simulink model "CthulhuFinalSimulation"  (R2019a)
settings: Solver=FixedStepDiscrete  StartTime=0.0  StopTime=500  FixedStep=dt  RelTol=1e-3
InitFcn:
  | clc
  | clear
  | 
  | timedelay = 0.05; %input lag, s
  | 
  | m = 2.5;
  | I = [0.034,  0.00008985,      -0.004;
  |         0.00008985,       0.075, -0.00000266;
  |       -0.004, -0.00000266,       0.102]; %kg m^2
  | 
  | L_p = 0.54; %length of pontoon, m
  | d_p = 0.1; %diameter of pontoon, m
  | V_p = 0.002536; %volume of pontoon, m
  | w_c = 0.347; %distance between pontoons, m
  | Zcm = 0.0; %height of cm wrt pontoons, m
  | 
  | wave_amp = 0.005; %amplitude of waves, m
  | f = 1.5; %freq of waves, Hz
  | 
  | Ayz = 0.002; %Area projected onto yz plane
  | Axz = 0.002; %Area projected onto xz plane
  | Axy = 0.005; %Area projected onto xy plane
  | Cdx = 2.2;
  | Cdy = 2.2;
  | Cdz = 2.2;
  | 
  | Iinv = I^-1;
  | dt = 0.005;
  | dtsim = 1/25;
  | dtdata = 0.01;
  | dtcontrol = 0.1;
  | timeseed = clock;
  | timeseed = round(timeseed(6));
  | wo = [0;0;0];
  | Ho = [0;0;0];
  | ro = [63;-31.5;d_p/2+0.3];
  | vo = [0;0;0];
  | qTarget = [1;0;0;0];
  | R = 0.1;
  | P = 0.0001;
  | Y = 0;
  | qo = [cos(R/2)*cos(P/2)*cos(Y/2)-sin(R/2)*sin(P/2)*sin(Y/2);
  |          sin(R/2)*cos(P/2)*cos(Y/2)+cos(R/2)*sin(P/2)*sin(Y/2);
  |          cos(R/2)*sin(P/2)*cos(Y/2)-sin(R/2)*cos(P/2)*sin(Y/2);
  |          sin(R/2)*sin(P/2)*cos(Y/2)+cos(R/2)*cos(P/2)*sin(Y/2)];
  | 
  | g = 9.80248;
  | rho = 997;
  | 
  | myworld = vrworld('CthulhuAssembly.wrl');
  | open(myworld);
  | set(0,'Units','pixels');
  | scnsize = get(0,'ScreenSize');
  | f1 = vrfigure(myworld,[1 80 scnsize(3)/2 scnsize(4)/2]);
  | set(f1,'Viewpoint','BodyView')
  | 
  | %pause(10)
StopFcn:
  | %plots_manual_control
undefined symbols (not defined in the file or in its folder): DiscIntNeverNeededParam
libraries: sharedtransform x5, vrlib x5, aerolibutil x3, aerolibanimutils x1, simulink x1
settings Model: Creator=washickb  LastModifiedBy=underwj5
settings DataIOCC: ReturnWorkspaceOutputs=off
settings DebuggingCC: ArithmeticOperatorsInVariantConditions=warning
settings SFSimCC: SimUseLocalCustomCode=off
settings RTWCC: RTWUseLocalCustomCode=off

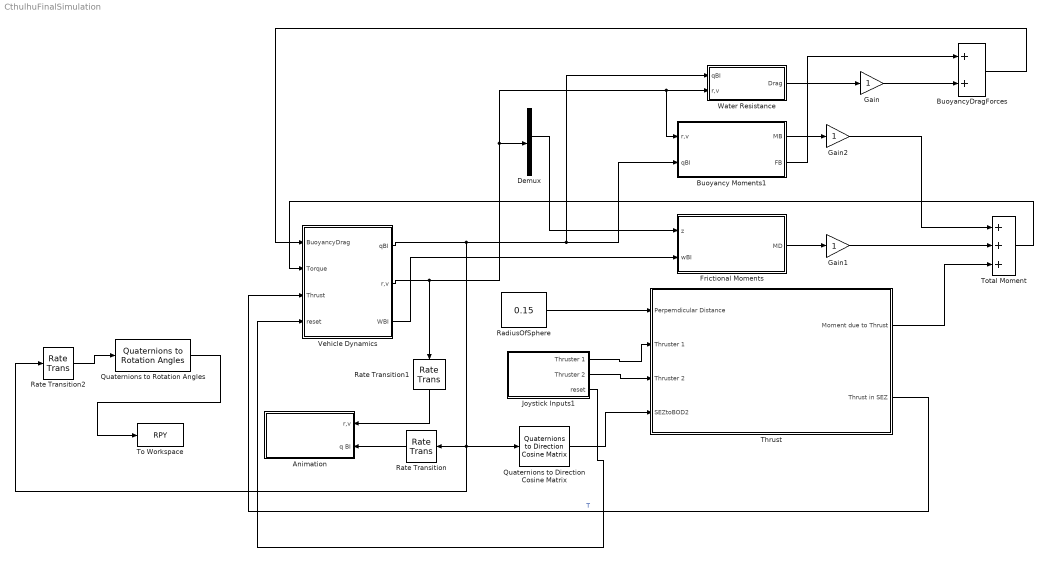
== system CthulhuFinalSimulation ==
  Animation : Subsystem
  Buoyancy Moments1 : Subsystem
  BuoyancyDragForces : Sum  Inputs=2
  Demux : Demux  Outputs=6
  Frictional Moments : Subsystem
  Gain : Gain
  Gain1 : Gain
  Gain2 : Gain
  Joystick Inputs1 : Subsystem
  Quaternions to Direction Cosine Matrix : sharedtransform/Quaternions to  Direction Cosine Matrix  aMode=aMode
      settings: SourceProductName=Aerospace Blockset  SourceProductBaseCode=AE
  Quaternions to Rotation Angles : sharedtransform/Quaternions to Rotation Angles  rotationOrder=XYZ  aMode=aMode
      settings: SourceProductBaseCode=AE
  RadiusOfSphere : Constant  Value=0.15
  Rate Transition : RateTransition  InitialCondition=qo  OutPortSampleTime=dtsim
  Rate Transition1 : RateTransition  InitialCondition=[ro;vo]  OutPortSampleTime=dtsim
  Rate Transition2 : RateTransition  InitialCondition=qo  OutPortSampleTime=dtdata
  "Thrust " : Subsystem
  To Workspace : ToWorkspace  VariableName=RPY  SaveFormat=Structure With Time  SampleTime=-1
  Total Moment : Sum  Inputs=+++
  Vehicle Dynamics : Subsystem
  Water Resistance : Subsystem
  wires:
  Vehicle Dynamics/2(r,v) -> Demux/1, Buoyancy Moments1/1(r,v), Water Resistance/2(r,v), Rate Transition1/1
  Vehicle Dynamics/1(qBI) -> Quaternions to Direction Cosine Matrix/1, Rate Transition2/1, Rate Transition/1, Water Resistance/1(qBI), Buoyancy Moments1/2(qBI)
  Rate Transition1/1 -> Animation/1(r,v)
  Rate Transition/1 -> Animation/2(q BI)
  Quaternions to Direction Cosine Matrix/1 -> "Thrust "/4(SEZtoBOD2)
  "Thrust "/1("Moment due to Thrust ") -> Total Moment/3
  Joystick Inputs1/2(Thruster 2) -> "Thrust "/3(Thruster 2)
  Joystick Inputs1/1(Thruster 1) -> "Thrust "/2(Thruster 1)
  RadiusOfSphere/1 -> "Thrust "/1(Perpemdicular Distance)
  Quaternions to Rotation Angles/1 -> To Workspace/1
  Vehicle Dynamics/3(WBI) -> Frictional Moments/2(wBI)
  Rate Transition2/1 -> Quaternions to Rotation Angles/1
  Total Moment/1 -> Vehicle Dynamics/2(Torque)
  "Thrust "/2(Thrust in SEZ) -> Vehicle Dynamics/3(Thrust)  "T"
  Buoyancy Moments1/1(MB) -> Gain2/1
  Demux/3 -> Frictional Moments/1(z)
  Frictional Moments/1("MD ") -> Gain1/1
  Water Resistance/1(Drag) -> Gain/1
  BuoyancyDragForces/1 -> Vehicle Dynamics/1(BuoyancyDrag)
  Gain/1 -> BuoyancyDragForces/2
  Gain1/1 -> Total Moment/2
  Gain2/1 -> Total Moment/1
  Buoyancy Moments1/2(FB) -> BuoyancyDragForces/1
  Joystick Inputs1/3(reset) -> Vehicle Dynamics/4(reset)

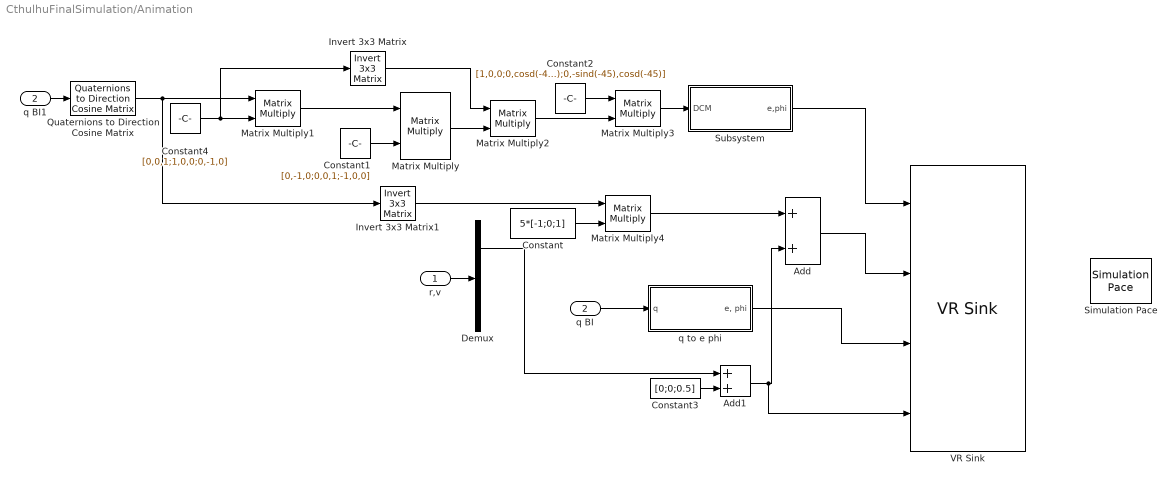
== system CthulhuFinalSimulation/Animation ==
  r,v : Inport
  q BI : Inport  Port=2
  Add : Sum
  Add1 : Sum
  Constant : Constant  Value=5*[-1;0;1]
  Constant1 : Constant  Value=[0,-1,0;0,0,1;-1,0,0]
  Constant2 : Constant  Value=[1,0,0;0,cosd(-45),sind(-45);0,-sind(-45),cosd(-45)]
  Constant3 : Constant  Value=[0;0;0.5]
  Constant4 : Constant  Value=[0,0,1;1,0,0;0,-1,0]
  Demux : Demux  Outputs=[3 3]
  Invert 3x3 Matrix : aerolibutil/Invert  3x3 Matrix
  Invert 3x3 Matrix1 : aerolibutil/Invert  3x3 Matrix
  Matrix Multiply{,1..4} (5 alike) : Product  Multiplication=Matrix(*)
  Quaternions to Direction Cosine Matrix : sharedtransform/Quaternions to  Direction Cosine Matrix  aMode=aMode
      settings: SourceProductName=Aerospace Blockset  SourceProductBaseCode=AE
  Simulation Pace : aerolibanimutils/Simulation Pace  SimulationPace=1  SleepMode=Auto  OutputPaceError=off  SampleTime=dt
  Subsystem : Subsystem
  VR Sink : vrlib/VR Sink  InstantiateOnLoad=on  SampleTime=0.1  ViewEnable=on  RemoteChange=off  RemoteView=off  FieldsWritten=BodyView.orientation.4.1.1.double#BodyView.position.3.1.1.double#Cthulhu.rotation.4.1.1.double#Cthulhu.translation.3.1.1.double  WorldFileName=CthulhuAssembly.wrl  AutoView=off  VideoDimensions=[]  AllowVariableSize=off
      settings: SourceProductName=Simulink
  q BI1 : InportShadow  Port=2
  q to e phi : Subsystem
  wires:
  r,v/1 -> Demux/1
  q BI/1 -> q to e phi/1("q ")
  Demux/1 -> Add1/1
  Constant1/1 -> Matrix Multiply/2
  Quaternions to Direction Cosine Matrix/1 -> Invert 3x3 Matrix1/1, Matrix Multiply1/1
  Add1/1 -> VR Sink/4, Add/2
  Constant3/1 -> Add1/2
  Constant/1 -> Matrix Multiply4/2
  q BI1/1 -> Quaternions to Direction Cosine Matrix/1
  Matrix Multiply2/1 -> Matrix Multiply3/2
  Matrix Multiply1/1 -> Matrix Multiply/1
  Constant4/1 -> Invert 3x3 Matrix/1, Matrix Multiply1/2
  Matrix Multiply/1 -> Matrix Multiply2/2
  Invert 3x3 Matrix/1 -> Matrix Multiply2/1
  Constant2/1 -> Matrix Multiply3/1
  Matrix Multiply3/1 -> Subsystem/1(DCM)
  Matrix Multiply4/1 -> Add/1
  Invert 3x3 Matrix1/1 -> Matrix Multiply4/1
  Subsystem/1(e,phi) -> VR Sink/1
  Add/1 -> VR Sink/2
  q to e phi/1("e, phi") -> VR Sink/3

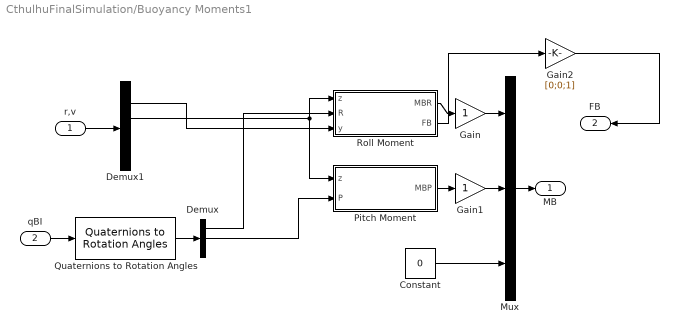
== system CthulhuFinalSimulation/Buoyancy Moments1 ==
  r,v : Inport
  qBI : Inport  Port=2
  Constant : Constant  Value=0
  Demux : Demux  Outputs=3
  Demux1 : Demux  Outputs=6
  Gain : Gain
  Gain1 : Gain
  Gain2 : Gain  Gain=[0;0;1]
  Mux : Mux  Inputs=3
  Pitch Moment : Subsystem
  Quaternions to Rotation Angles : sharedtransform/Quaternions to Rotation Angles  rotationOrder=XYZ  aMode=aMode
      settings: SourceProductBaseCode=AE
  Roll Moment : Subsystem
  MB : Outport
  FB : Outport  Port=2
  wires:
  Constant/1 -> Mux/3
  Mux/1 -> MB/1
  Pitch Moment/1(MBP) -> Gain1/1
  Roll Moment/1(MBR) -> Gain/1
  qBI/1 -> Quaternions to Rotation Angles/1
  Quaternions to Rotation Angles/1 -> Demux/1
  Demux/1 -> Roll Moment/2(R)
  Demux/2 -> Pitch Moment/2(P)
  Gain/1 -> Mux/1
  Gain1/1 -> Mux/2
  Roll Moment/2(FB) -> Gain2/1
  Gain2/1 -> FB/1
  r,v/1 -> Demux1/1
  Demux1/3 -> Pitch Moment/1(z), Roll Moment/1(z)
  Demux1/2 -> Roll Moment/3(y)

== system CthulhuFinalSimulation/Frictional Moments ==
  z : Inport
  wBI : Inport  Port=2
  Add : Sum  Inputs=+---
  Constant : Constant  Value=Zcm
  Constant1 : Constant  Value=d_p/2
  Constant2 : Constant  Value=.05
  If : If  IfExpression=u1 < 0
  If Action Subsystem : Subsystem  TreatAsAtomicUnit=on
  Merge : Merge
  Subsystem : Subsystem
  "MD " : Outport
  wires:
  If/1 -> Subsystem/Action  "z<d_p"
  If/2 -> If Action Subsystem/Action
  Subsystem/1(MD) -> Merge/2
  If Action Subsystem/1(Out1) -> Merge/1
  Merge/1 -> "MD "/1
  z/1 -> Add/1
  Constant/1 -> Add/2
  Constant1/1 -> Add/3
  Add/1 -> If/1
  Constant2/1 -> Add/4
  wBI/1 -> Subsystem/1(wBI)

== system CthulhuFinalSimulation/Joystick Inputs1 ==
  Demux : Demux  Outputs=5
  Demux1 : Demux  Outputs=10
  Gain1 : Gain  Gain=-1
  Gain2 : Gain  Gain=-1
  Joystick Input : vrlib/Joystick Input  joyid=1  adjustports=on  forcefeed=off
      settings: SourceProductName=Simulink
  Stop Simulation : Stop
  Subsystem : Subsystem
  Subsystem2 : Subsystem
  Thruster 1 : Outport
  Thruster 2 : Outport  Port=2
  reset : Outport  Port=3
  wires:
  Demux/2 -> Gain1/1
  Gain1/1 -> Subsystem/1(pad y)  "pad y"
  Joystick Input/1 -> Demux/1
  Gain2/1 -> Subsystem2/1(pad y)  "pad y"
  Demux/5 -> Gain2/1
  Subsystem2/1(thrust) -> Thruster 2/1
  Subsystem/1(thrust) -> Thruster 1/1
  Joystick Input/2 -> Demux1/1
  Demux1/8 -> reset/1
  Demux1/1 -> Stop Simulation/1

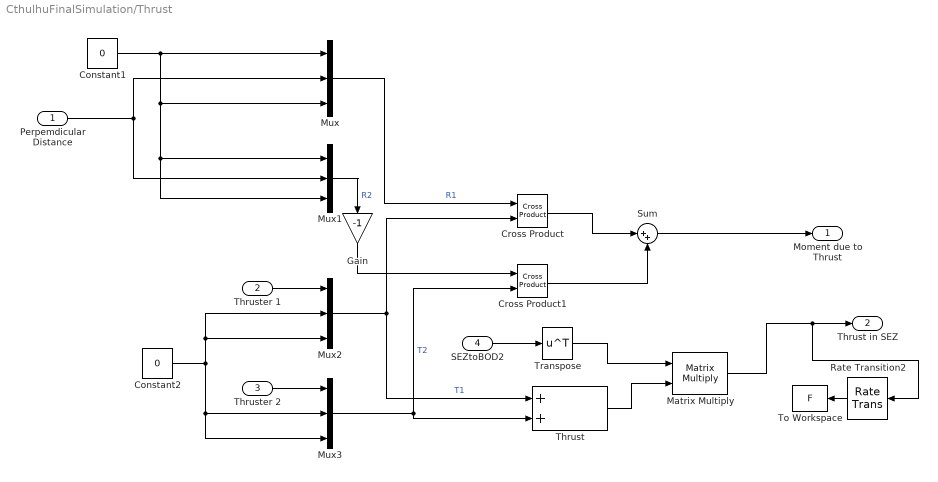
== system CthulhuFinalSimulation/Thrust  ==
  Perpemdicular Distance : Inport
  Thruster 1 : Inport  Port=2
  Thruster 2 : Inport  Port=3
  SEZtoBOD2 : Inport  Port=4
  Constant1 : Constant  Value=0
  Constant2 : Constant  Value=0
  Cross Product : vrlib/Utilities/Cross Product
      settings: SourceProductName=Simulink
  Cross Product1 : vrlib/Utilities/Cross Product
      settings: SourceProductName=Simulink
  Gain : Gain  Gain=-1
  Matrix Multiply : Product  Multiplication=Matrix(*)
  Mux{,1..3} (4 alike) : Mux  Inputs=3
  Rate Transition2 : RateTransition  InitialCondition=[0;0;0]  OutPortSampleTime=dtdata
  Sum : Sum  Inputs=|++
  Thrust : Sum  Inputs=2
  To Workspace : ToWorkspace  VariableName=F  SaveFormat=Structure With Time  SampleTime=-1
  Transpose : Math  Operator=transpose  SaturateOnIntegerOverflow=on
  "Moment due to Thrust " : Outport
  Thrust in SEZ : Outport  Port=2
  wires:
  Perpemdicular Distance/1 -> Mux1/2, Mux/2
  Constant1/1 -> Mux/1, Mux1/3, Mux1/1, Mux/3
  Thruster 1/1 -> Mux2/1
  Thruster 2/1 -> Mux3/1
  Constant2/1 -> Mux3/3, Mux3/2, Mux2/3, Mux2/2
  Mux2/1 -> Cross Product/2, Thrust/1  "T1"
  Mux3/1 -> Cross Product1/2, Thrust/2  "T2"
  Mux/1 -> Cross Product/1  "R1"
  Mux1/1 -> Gain/1  "R2"
  Cross Product/1 -> Sum/1
  Cross Product1/1 -> Sum/2
  Sum/1 -> "Moment due to Thrust "/1
  SEZtoBOD2/1 -> Transpose/1
  Transpose/1 -> Matrix Multiply/1
  Thrust/1 -> Matrix Multiply/2
  Matrix Multiply/1 -> Rate Transition2/1, Thrust in SEZ/1
  Gain/1 -> Cross Product1/1
  Rate Transition2/1 -> To Workspace/1

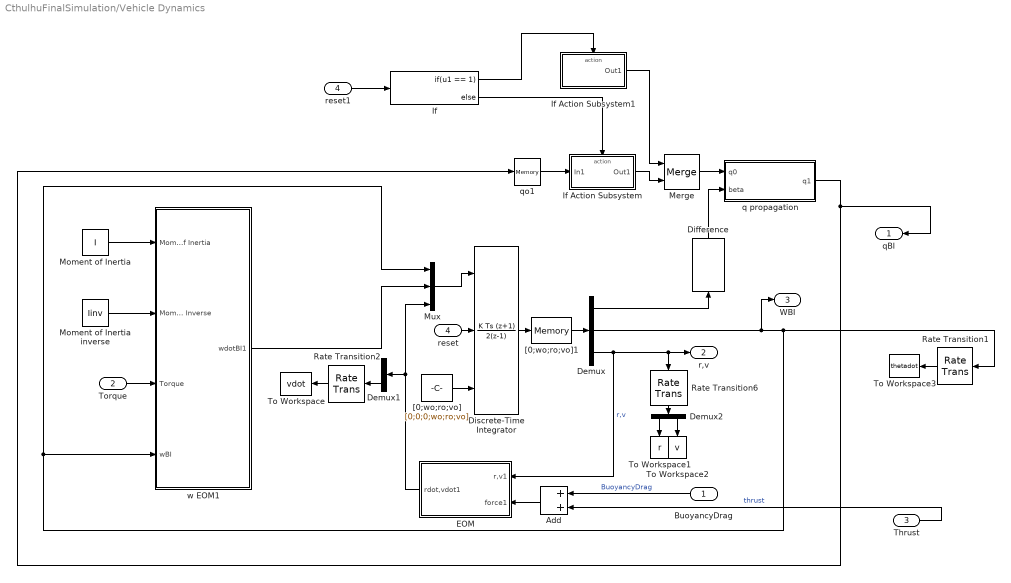
== system CthulhuFinalSimulation/Vehicle Dynamics ==
  BuoyancyDrag : Inport
  Torque : Inport  Port=2
  Thrust : Inport  Port=3
  reset : Inport  Port=4
  Add : Sum
  Demux : Demux  Outputs=[3 3 6]
  Demux1 : Demux  Outputs=2
  Demux2 : Demux  Outputs=2
  Difference : simulink/Discrete/Difference  ICPrevInput=0.0  OutMin=[]  OutMax=[]  OutDataType=fixdt(1, 16)  OutScaling=2^-10  DoSatur=off
  Discrete-Time Integrator : DiscreteIntegrator  IntegratorMethod=Integration: Trapezoidal  ExternalReset=rising  InitialConditionSource=external  SampleTime=dt  ICPrevOutput=DiscIntNeverNeededParam  ICPrevScaledInput=DiscIntNeverNeededParam
  EOM : Subsystem
  If : If  IfExpression=u1 == 1
  If Action Subsystem : Subsystem  TreatAsAtomicUnit=on
  If Action Subsystem1 : Subsystem  TreatAsAtomicUnit=on
  Merge : Merge
  Moment of Inertia : Constant  Value=I
  Moment of Inertia inverse : Constant  Value=Iinv
  Mux : Mux  Inputs=3
  Rate Transition1 : RateTransition  InitialCondition=[0;0;0]  OutPortSampleTime=dtdata
  Rate Transition2 : RateTransition  InitialCondition=[0;0;0]  OutPortSampleTime=dtdata
  Rate Transition6 : RateTransition  InitialCondition=[0;0;0;0;0;0]  OutPortSampleTime=dtdata
  To Workspace : ToWorkspace  VariableName=vdot  SaveFormat=Structure With Time  SampleTime=-1
  To Workspace1 : ToWorkspace  VariableName=r  SaveFormat=Structure With Time  SampleTime=-1
  To Workspace2 : ToWorkspace  VariableName=v  SaveFormat=Structure With Time  SampleTime=-1
  To Workspace3 : ToWorkspace  VariableName=thetadot  SaveFormat=Structure With Time  SampleTime=-1
  "[0;wo;ro;vo]" : Constant  Value=[0;0;0;wo;ro;vo]
  "[0;wo;ro;vo]1" : Memory  InitialCondition=[0;0;0;wo;ro;vo]  InheritSampleTime=on
  q propagation : Subsystem
  qo1 : Memory  InitialCondition=qo
  reset1 : InportShadow  Port=4
  w EOM1 : Subsystem
  qBI : Outport
  r,v : Outport  Port=2
  WBI : Outport  Port=3
  wires:
  Difference/1 -> q propagation/2(beta)
  Moment of Inertia/1 -> w EOM1/1(Moment of Inertia)
  Moment of Inertia inverse/1 -> w EOM1/2(Moment of Inertia Inverse)
  qo1/1 -> If Action Subsystem/1(In1)
  Discrete-Time Integrator/1 -> "[0;wo;ro;vo]1"/1
  Mux/1 -> Discrete-Time Integrator/1
  Demux/3 -> EOM/1(r,v1), r,v/1, Rate Transition6/1  "r,v"
  "[0;wo;ro;vo]1"/1 -> Demux/1
  q propagation/1(q1) -> qo1/1, qBI/1
  Torque/1 -> w EOM1/3(Torque)
  "[0;wo;ro;vo]"/1 -> Discrete-Time Integrator/3
  Demux/1 -> Difference/1
  w EOM1/1(wdotBI1) -> Mux/2
  Demux1/2 -> Rate Transition2/1
  Rate Transition2/1 -> To Workspace/1
  EOM/1(rdot,vdot1) -> Demux1/1, Mux/3
  Thrust/1 -> Add/2  "thrust"
  BuoyancyDrag/1 -> Add/1  "BuoyancyDrag"
  Rate Transition6/1 -> Demux2/1
  Demux2/1 -> To Workspace1/1
  Demux2/2 -> To Workspace2/1
  Add/1 -> EOM/2(force1)
  Demux/2 -> Rate Transition1/1, w EOM1/4(wBI), Mux/1, WBI/1
  Rate Transition1/1 -> To Workspace3/1
  reset/1 -> Discrete-Time Integrator/2
  reset1/1 -> If/1
  If/2 -> If Action Subsystem/Action
  If/1 -> If Action Subsystem1/Action
  Merge/1 -> q propagation/1(q0)
  If Action Subsystem1/1(Out1) -> Merge/1
  If Action Subsystem/1(Out1) -> Merge/2

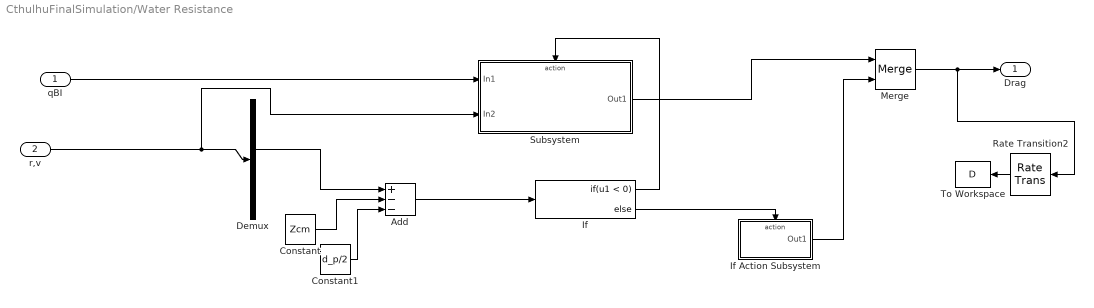
== system CthulhuFinalSimulation/Water Resistance ==
  qBI : Inport
  r,v : Inport  Port=2
  Add : Sum  Inputs=+--
  Constant : Constant  Value=Zcm
  Constant1 : Constant  Value=d_p/2
  Demux : Demux  Outputs=6
  If : If  IfExpression=u1 < 0
  If Action Subsystem : Subsystem  TreatAsAtomicUnit=on
  Merge : Merge
  Rate Transition2 : RateTransition  InitialCondition=[0;0;0]  OutPortSampleTime=dtdata
  Subsystem : Subsystem
  To Workspace : ToWorkspace  VariableName=D  SaveFormat=Structure With Time  SampleTime=-1
  Drag : Outport
  wires:
  qBI/1 -> Subsystem/1(In1)
  r,v/1 -> Subsystem/2(In2), Demux/1
  Constant/1 -> Add/2
  Constant1/1 -> Add/3
  Demux/3 -> Add/1
  Add/1 -> If/1
  If/1 -> Subsystem/Action
  If/2 -> If Action Subsystem/Action
  If Action Subsystem/1(Out1) -> Merge/2
  Subsystem/1(Out1) -> Merge/1
  Merge/1 -> Rate Transition2/1, Drag/1
  Rate Transition2/1 -> To Workspace/1

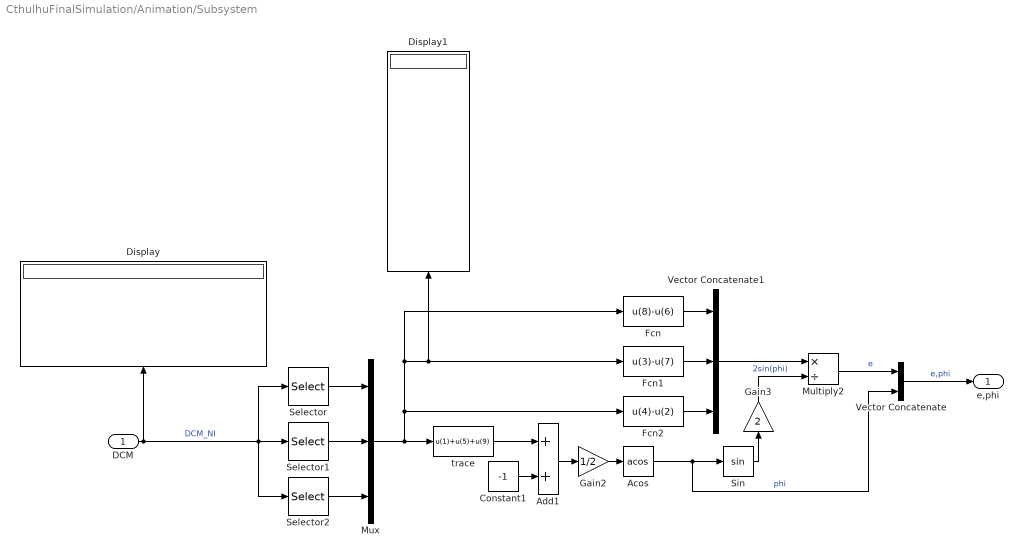
== system CthulhuFinalSimulation/Animation/Subsystem ==
  DCM : Inport
  Acos : Trigonometry  Operator=acos
  Add1 : Sum
  Constant1 : Constant  Value=-1
  Display : Display
  Display1 : Display
  Fcn : Fcn  Expr=u(8)-u(6)
  Fcn1 : Fcn  Expr=u(3)-u(7)
  Fcn2 : Fcn  Expr=u(4)-u(2)
  Gain2 : Gain  Gain=1/2
  Gain3 : Gain  Gain=2
  Multiply2 : Product  Inputs=*/
  Mux : Mux  Inputs=3
  Selector : Selector  NumberOfDimensions=2  InputPortWidth=3  IndexOptions=Select all,Index vector (dialog)  Indices=[1 3],1  OutputSizes=1,1
  Selector1 : Selector  NumberOfDimensions=2  InputPortWidth=3  IndexOptions=Select all,Index vector (dialog)  Indices=[1 3],2  OutputSizes=1,1
  Selector2 : Selector  NumberOfDimensions=2  InputPortWidth=3  IndexOptions=Select all,Index vector (dialog)  Indices=[1 3],3  OutputSizes=1,1
  Sin : Trigonometry
  Vector Concatenate : Concatenate
  Vector Concatenate1 : Concatenate  NumInputs=3
  trace : Fcn  Expr=u(1)+u(5)+u(9)
  e,phi : Outport
  wires:
  Vector Concatenate1/1 -> Multiply2/1
  trace/1 -> Add1/1
  Add1/1 -> Gain2/1
  Vector Concatenate/1 -> e,phi/1  "e,phi"
  Constant1/1 -> Add1/2
  Fcn/1 -> Vector Concatenate1/1
  Gain3/1 -> Multiply2/2  "2sin(phi)"
  Multiply2/1 -> Vector Concatenate/1  "e"
  Sin/1 -> Gain3/1
  Fcn1/1 -> Vector Concatenate1/2
  Acos/1 -> Vector Concatenate/2, Sin/1  "phi"
  Fcn2/1 -> Vector Concatenate1/3
  Gain2/1 -> Acos/1
  Mux/1 -> Fcn2/1, Fcn1/1, Display1/1, Fcn/1, trace/1
  Selector/1 -> Mux/1
  Selector1/1 -> Mux/2
  Selector2/1 -> Mux/3
  DCM/1 -> Selector2/1, Selector/1, Selector1/1, Display/1  "DCM_NI"

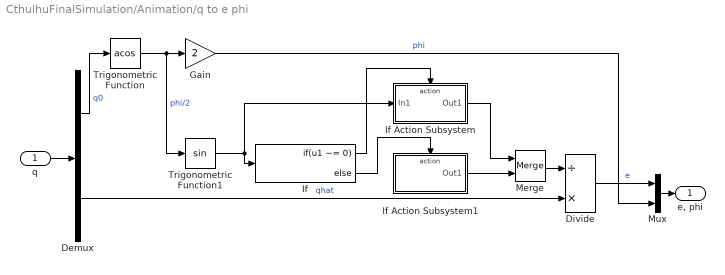
== system CthulhuFinalSimulation/Animation/q to e phi ==
  "q " : Inport
  Demux : Demux  Outputs=[1,3]
  Divide : Product  Inputs=/*
  Gain : Gain  Gain=2
  If : If  IfExpression=u1 ~= 0
  If Action Subsystem : Subsystem  TreatAsAtomicUnit=on
  If Action Subsystem1 : Subsystem  TreatAsAtomicUnit=on
  Merge : Merge
  Mux : Mux  Inputs=2
  Trigonometric Function : Trigonometry  Operator=acos
  Trigonometric Function1 : Trigonometry
  "e, phi" : Outport
  wires:
  Gain/1 -> Mux/2  "phi"
  Demux/1 -> Trigonometric Function/1  "q0"
  Trigonometric Function1/1 -> If/1, If Action Subsystem/1(In1)
  Divide/1 -> Mux/1  "e"
  Trigonometric Function/1 -> Trigonometric Function1/1, Gain/1  "phi/2"
  Mux/1 -> "e, phi"/1
  Demux/2 -> Divide/2  "qhat"
  "q "/1 -> Demux/1
  If/1 -> If Action Subsystem/Action
  If/2 -> If Action Subsystem1/Action
  If Action Subsystem/1(Out1) -> Merge/1
  If Action Subsystem1/1(Out1) -> Merge/2
  Merge/1 -> Divide/1

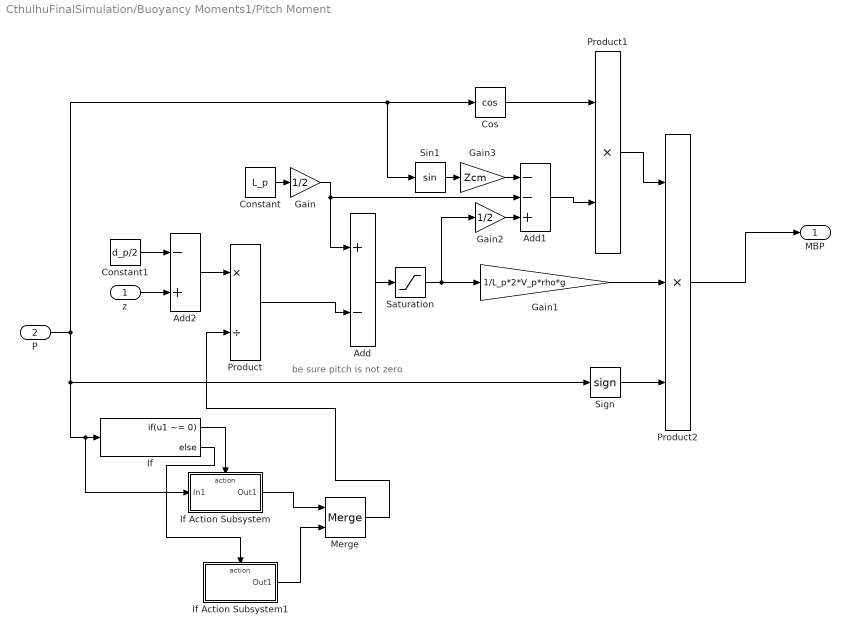
== system CthulhuFinalSimulation/Buoyancy Moments1/Pitch Moment ==
  note: be sure pitch is not zero
  z : Inport
  P : Inport  Port=2
  Add : Sum  Inputs=+-
  Add1 : Sum  Inputs=--+
  Add2 : Sum  Inputs=-+
  Constant : Constant  Value=L_p
  Constant1 : Constant  Value=d_p/2
  Cos : Trigonometry  Operator=cos
  Gain : Gain  Gain=1/2
  Gain1 : Gain  Gain=1/L_p*2*V_p*rho*g
  Gain2 : Gain  Gain=1/2
  Gain3 : Gain  Gain=Zcm
  If : If  IfExpression=u1 ~= 0
  If Action Subsystem : Subsystem  TreatAsAtomicUnit=on
  If Action Subsystem1 : Subsystem  TreatAsAtomicUnit=on
  Merge : Merge
  Product : Product  Inputs=*/
  Product1 : Product
  Product2 : Product  Inputs=3
  Saturation : Saturate  UpperLimit=L_p  LowerLimit=0
  Sign : Signum
  Sin1 : Trigonometry
  MBP : Outport
  wires:
  Constant/1 -> Gain/1
  P/1 -> If Action Subsystem/1(In1), If/1, Sign/1, Sin1/1, Cos/1
  If Action Subsystem/1(Out1) -> Merge/1
  z/1 -> Add2/2
  Gain/1 -> Add1/2, Add/1
  Add/1 -> Saturation/1
  Gain2/1 -> Add1/3
  Add1/1 -> Product1/2
  Cos/1 -> Product1/1
  Product1/1 -> Product2/1
  Gain1/1 -> Product2/2
  Product2/1 -> MBP/1
  Saturation/1 -> Gain2/1, Gain1/1
  Sign/1 -> Product2/3
  Constant1/1 -> Add2/1
  Add2/1 -> Product/1
  Gain3/1 -> Add1/1
  Sin1/1 -> Gain3/1
  If/1 -> If Action Subsystem/Action
  If/2 -> If Action Subsystem1/Action
  If Action Subsystem1/1(Out1) -> Merge/2
  Merge/1 -> Product/2
  Product/1 -> Add/2

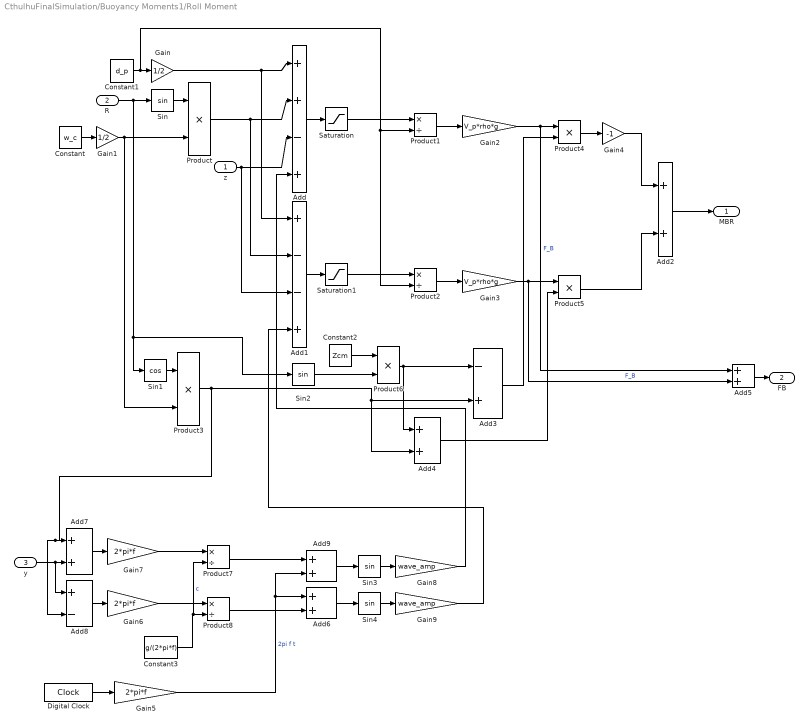
== system CthulhuFinalSimulation/Buoyancy Moments1/Roll Moment ==
  z : Inport
  R : Inport  Port=2
  y : Inport  Port=3
  Add : Sum  Inputs=++-+
  Add1 : Sum  Inputs=+--+
  Add{2,4..7,9} (6 alike) : Sum
  Add3 : Sum  Inputs=-+
  Add8 : Sum  Inputs=+-
  Constant : Constant  Value=w_c
  Constant1 : Constant  Value=d_p
  Constant2 : Constant  Value=Zcm
  Constant3 : Constant  Value=g/(2*pi*f)
  Digital Clock : DigitalClock  SampleTime=dt
  Gain : Gain  Gain=1/2
  Gain1 : Gain  Gain=1/2
  Gain2 : Gain  Gain=V_p*rho*g
  Gain3 : Gain  Gain=V_p*rho*g
  Gain4 : Gain  Gain=-1
  Gain5 : Gain  Gain=2*pi*f
  Gain6 : Gain  Gain=2*pi*f
  Gain7 : Gain  Gain=2*pi*f
  Gain8 : Gain  Gain=wave_amp
  Gain9 : Gain  Gain=wave_amp
  Product{,3..6} (5 alike) : Product
  Product{1..2,7..8} (4 alike) : Product  Inputs=*/
  Saturation : Saturate  UpperLimit=d_p  LowerLimit=0
  Saturation1 : Saturate  UpperLimit=d_p  LowerLimit=0
  Sin{,2..4} (4 alike) : Trigonometry
  Sin1 : Trigonometry  Operator=cos
  MBR : Outport
  FB : Outport  Port=2
  wires:
  Constant1/1 -> Product2/2, Product1/2, Gain/1
  Constant/1 -> Gain1/1
  R/1 -> Sin/1, Sin2/1, Sin1/1
  Gain/1 -> Add1/1, Add/1
  Sin/1 -> Product/1
  Gain1/1 -> Product3/2, Product/2
  Product/1 -> Add1/2, Add/2
  z/1 -> Add1/3, Add/3
  Add/1 -> Saturation/1
  Add1/1 -> Saturation1/1
  Saturation/1 -> Product1/1
  Saturation1/1 -> Product2/1
  Product1/1 -> Gain2/1
  Product2/1 -> Gain3/1
  Sin1/1 -> Product3/1
  Gain2/1 -> Add5/1, Product4/1  "F_B"
  Gain3/1 -> Add5/2, Product5/1  "F_B"
  Add3/1 -> Product4/2
  Product4/1 -> Gain4/1
  Gain4/1 -> Add2/1
  Product5/1 -> Add2/2
  Add2/1 -> MBR/1
  Constant2/1 -> Product6/1
  Product6/1 -> Add4/1, Add3/1
  Sin2/1 -> Product6/2
  Add4/1 -> Product5/2
  Add5/1 -> FB/1
  Digital Clock/1 -> Gain5/1
  Gain5/1 -> Add6/1, Add9/2  "2pi f t"
  Product3/1 -> Add8/2, Add7/1, Add4/2, Add3/2
  y/1 -> Add8/1, Add7/2
  Add7/1 -> Gain7/1
  Add8/1 -> Gain6/1
  Gain6/1 -> Product8/1
  Gain7/1 -> Product7/1
  Add9/1 -> Sin3/1
  Add6/1 -> Sin4/1
  Sin3/1 -> Gain8/1
  Sin4/1 -> Gain9/1
  Product8/1 -> Add6/2
  Product7/1 -> Add9/1
  Constant3/1 -> Product7/2, Product8/2  "c"
  Gain8/1 -> Add/4
  Gain9/1 -> Add1/4

== system CthulhuFinalSimulation/Frictional Moments/If Action Subsystem ==
  Action Port : ActionPort  ActionPortLabel=else
  Constant : Constant  Value=[0;0;0]
  Out1 : Outport
  wires:
  Constant/1 -> Out1/1

== system CthulhuFinalSimulation/Frictional Moments/Subsystem ==
  wBI : Inport
  Action Port : ActionPort  ActionPortLabel=if(u1 < 0)
  Demux : Demux  Outputs=3
  Gain1 : Gain  Gain=-10
  Gain2 : Gain  Gain=-10
  Gain3 : Gain  Gain=-3
  Mux : Mux  Inputs=3
  MD : Outport
  wires:
  Demux/1 -> Gain1/1  "wx"
  Demux/2 -> Gain2/1  "wy"
  Demux/3 -> Gain3/1  "wz"
  wBI/1 -> Demux/1
  Gain1/1 -> Mux/1
  Gain2/1 -> Mux/2
  Gain3/1 -> Mux/3
  Mux/1 -> MD/1

== system CthulhuFinalSimulation/Joystick Inputs1/Subsystem ==
  pad y : Inport
  If : If  IfExpression=u1 <= 0
  Merge : Merge
  throttle1 : Subsystem  TreatAsAtomicUnit=on
  throttle2 : Subsystem  TreatAsAtomicUnit=on
  thrust : Outport  VectorParamsAs1DForOutWhenUnconnected=on
  wires:
  If/2 -> throttle2/Action
  throttle2/1(ThrustPositive) -> Merge/2
  pad y/1 -> throttle2/1(In2), throttle1/1(In1), If/1
  throttle1/1(ThrustNegative) -> Merge/1
  If/1 -> throttle1/Action
  Merge/1 -> thrust/1

== system CthulhuFinalSimulation/Joystick Inputs1/Subsystem2 ==
  pad y : Inport
  If : If  IfExpression=u1 <= 0
  Merge : Merge
  throttle1 : Subsystem  TreatAsAtomicUnit=on
  throttle2 : Subsystem  TreatAsAtomicUnit=on
  thrust : Outport  VectorParamsAs1DForOutWhenUnconnected=on
  wires:
  If/2 -> throttle2/Action
  throttle2/1(ThrustPositive) -> Merge/2
  pad y/1 -> throttle2/1(In2), throttle1/1(In1), If/1
  throttle1/1(ThrustNegative) -> Merge/1
  If/1 -> throttle1/Action
  Merge/1 -> thrust/1

== system CthulhuFinalSimulation/Vehicle Dynamics/EOM ==
  r,v1 : Inport
  force1 : Inport  Port=2
  Constant4 : Constant  Value=0
  Constant5 : Constant  Value=0
  Constant6 : Constant  Value=-g
  Demux1 : Demux  Outputs=6
  Gain2 : Gain  Gain=1/m
  Mux4 : Mux  Inputs=3
  Mux5 : Mux  Inputs=2
  Mux6 : Mux  Inputs=3
  Sum : Sum  Inputs=|++
  rdot,vdot1 : Outport
  wires:
  force1/1 -> Gain2/1
  Constant6/1 -> Mux4/3  "zddot"
  r,v1/1 -> Demux1/1
  Demux1/5 -> Mux6/2  "ydot"
  Mux6/1 -> Mux5/1  "rdot"
  Constant4/1 -> Mux4/1  "xddot"
  Constant5/1 -> Mux4/2  "yddot"
  Demux1/6 -> Mux6/3  "zdot"
  Mux5/1 -> rdot,vdot1/1
  Demux1/4 -> Mux6/1  "xdot"
  Mux4/1 -> Sum/1
  Gain2/1 -> Sum/2
  Sum/1 -> Mux5/2  "vdot"

== system CthulhuFinalSimulation/Vehicle Dynamics/If Action Subsystem ==
  In1 : Inport
  Action Port : ActionPort  ActionPortLabel=else
  Out1 : Outport
  wires:
  In1/1 -> Out1/1

== system CthulhuFinalSimulation/Vehicle Dynamics/If Action Subsystem1 ==
  Action Port : ActionPort  ActionPortLabel=if(u1 == 1)
  Constant : Constant  Value=qo
  Out1 : Outport
  wires:
  Constant/1 -> Out1/1

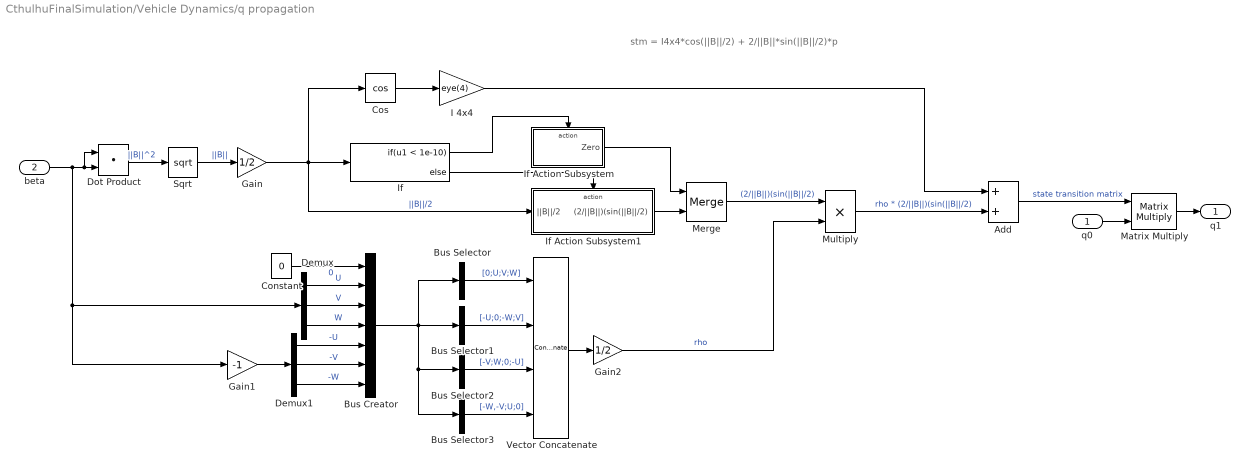
== system CthulhuFinalSimulation/Vehicle Dynamics/q propagation ==
  note: stm = I4x4*cos(||B||/2) + 2/||B||*sin(||B||/2)*p
  q0 : Inport  PortDimensions=[4,1]
  beta : Inport  Port=2
  Add : Sum
  Bus Creator : BusCreator  Inputs=7
  Bus Selector : BusSelector  OutputSignals=0,U,V,W  OutputAsBus=on
  Bus Selector1 : BusSelector  OutputSignals=-U,0,-W,V  OutputAsBus=on
  Bus Selector2 : BusSelector  OutputSignals=-V,W,0,-U  OutputAsBus=on
  Bus Selector3 : BusSelector  OutputSignals=-W,-V,U,0  OutputAsBus=on
  Constant : Constant  Value=0
  Cos : Trigonometry  Operator=cos
  Demux : Demux  Outputs=3
  Demux1 : Demux  Outputs=3
  Dot Product : DotProduct  InputSameDT=on  OutDataTypeStr=Inherit: Inherit via internal rule
  Gain : Gain  Gain=1/2
  Gain1 : Gain  Gain=-1
  Gain2 : Gain  Gain=1/2
  I 4x4 : Gain  Gain=eye(4)
  If : If  IfExpression=u1 < 1e-10
  If Action Subsystem : Subsystem  TreatAsAtomicUnit=on
  If Action Subsystem1 : Subsystem  TreatAsAtomicUnit=on
  Matrix Multiply : Product  Multiplication=Matrix(*)
  Merge : Merge
  Multiply : Product
  Sqrt : Sqrt  SaturateOnIntegerOverflow=on
  Vector Concatenate : Concatenate  NumInputs=4  Mode=Multidimensional array  ConcatenateDimension=2
  q1 : Outport
  wires:
  Gain/1 -> Cos/1, If Action Subsystem1/1(||B||/2), If/1  "||B||/2"
  If/2 -> If Action Subsystem1/Action
  If Action Subsystem/1(Zero) -> Merge/1
  If/1 -> If Action Subsystem/Action
  If Action Subsystem1/1((2/||B||)(sin(||B||/2)) -> Merge/2
  Merge/1 -> Multiply/1  "(2/||B||)(sin(||B||/2)"
  beta/1 -> Dot Product/1, Dot Product/2, Demux/1, Gain1/1
  q0/1 -> Matrix Multiply/2
  Matrix Multiply/1 -> q1/1
  Cos/1 -> I 4x4/1
  I 4x4/1 -> Add/1
  Add/1 -> Matrix Multiply/1  "state transition matrix"
  Gain1/1 -> Demux1/1
  Demux/1 -> Bus Creator/2  "U"
  Demux/2 -> Bus Creator/3  "V"
  Demux/3 -> Bus Creator/4  "W"
  Demux1/1 -> Bus Creator/5  "-U"
  Demux1/2 -> Bus Creator/6  "-V"
  Demux1/3 -> Bus Creator/7  "-W"
  Bus Creator/1 -> Bus Selector3/1, Bus Selector2/1, Bus Selector/1, Bus Selector1/1
  Constant/1 -> Bus Creator/1  "0"
  Bus Selector/1 -> Vector Concatenate/1  "[0;U;V;W]"
  Bus Selector1/1 -> Vector Concatenate/2  "[-U;0;-W;V]"
  Bus Selector2/1 -> Vector Concatenate/3  "[-V;W;0;-U]"
  Bus Selector3/1 -> Vector Concatenate/4  "[-W,-V;U;0]"
  Vector Concatenate/1 -> Gain2/1
  Multiply/1 -> Add/2  "rho * (2/||B||)(sin(||B||/2)"
  Gain2/1 -> Multiply/2  "rho"
  Dot Product/1 -> Sqrt/1  "||B||^2"
  Sqrt/1 -> Gain/1  "||B||"

== system CthulhuFinalSimulation/Vehicle Dynamics/w EOM1 ==
  note: wBIdot = I_inv*(T - wBI x ([I]wBI + Ho))
  Moment of Inertia : Inport
  Moment of Inertia Inverse : Inport  Port=2
  Torque : Inport  Port=3
  wBI : Inport  Port=4
  Add : Sum
  Cross Product : vrlib/Utilities/Cross Product
      settings: SourceProductBaseCode=VR
  Gain : Gain  Gain=-1
  Matrix Multiply : Product  Multiplication=Matrix(*)
  Matrix Multiply1 : Product  Multiplication=Matrix(*)
  wdotBI1 : Outport
  wires:
  Moment of Inertia/1 -> Matrix Multiply/1
  Matrix Multiply/1 -> Cross Product/2  "WI"
  Gain/1 -> Cross Product/1  "-w"
  Cross Product/1 -> Add/1  "-w x [I]w"
  Moment of Inertia Inverse/1 -> Matrix Multiply1/1
  Matrix Multiply1/1 -> wdotBI1/1  "wdotBI"
  Torque/1 -> Add/2
  Add/1 -> Matrix Multiply1/2
  wBI/1 -> Matrix Multiply/2, Gain/1  "wBI"

== system CthulhuFinalSimulation/Water Resistance/If Action Subsystem ==
  Action Port : ActionPort  ActionPortLabel=else
  Constant : Constant  Value=[0;0;0]
  Out1 : Outport
  wires:
  Constant/1 -> Out1/1

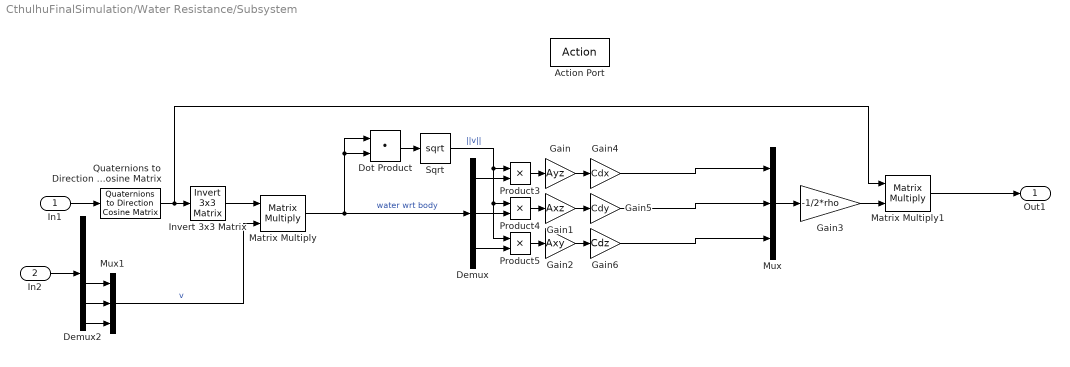
== system CthulhuFinalSimulation/Water Resistance/Subsystem ==
  In1 : Inport
  In2 : Inport  Port=2
  Action Port : ActionPort  ActionPortLabel=if(u1 < 0)
  Demux : Demux  Outputs=3
  Demux2 : Demux  Outputs=6
  Dot Product : DotProduct  InputSameDT=on  OutDataTypeStr=Inherit: Inherit via internal rule
  Gain : Gain  Gain=Ayz
  Gain1 : Gain  Gain=Axz
  Gain2 : Gain  Gain=Axy
  Gain3 : Gain  Gain=-1/2*rho
  Gain4 : Gain  Gain=Cdx
  Gain5 : Gain  Gain=Cdy
  Gain6 : Gain  Gain=Cdz
  Invert 3x3 Matrix : aerolibutil/Invert  3x3 Matrix
  Matrix Multiply : Product  Multiplication=Matrix(*)
  Matrix Multiply1 : Product  Multiplication=Matrix(*)
  Mux : Mux  Inputs=3
  Mux1 : Mux  Inputs=3
  Product3 : Product
  Product4 : Product
  Product5 : Product
  Quaternions to Direction Cosine Matrix : sharedtransform/Quaternions to  Direction Cosine Matrix  aMode=aMode
      settings: SourceProductName=Aerospace Blockset  SourceProductBaseCode=AE
  Sqrt : Sqrt  SaturateOnIntegerOverflow=on
  Out1 : Outport
  wires:
  Matrix Multiply/1 -> Demux/1, Dot Product/1, Dot Product/2  "water wrt body"
  Gain6/1 -> Mux/3
  Gain1/1 -> Gain5/1
  Gain4/1 -> Mux/1
  Mux/1 -> Gain3/1
  Gain5/1 -> Mux/2
  Demux/2 -> Product4/2
  Gain2/1 -> Gain6/1
  Mux1/1 -> Matrix Multiply/2  "v"
  Matrix Multiply1/1 -> Out1/1
  Gain/1 -> Gain4/1
  Product4/1 -> Gain1/1
  Sqrt/1 -> Product5/1, Product4/1, Product3/1  "||v||"
  In2/1 -> Demux2/1
  Demux/3 -> Product5/2
  Demux2/6 -> Mux1/3
  Product5/1 -> Gain2/1
  Dot Product/1 -> Sqrt/1
  Demux/1 -> Product3/2
  Gain3/1 -> Matrix Multiply1/2
  Demux2/5 -> Mux1/2
  Demux2/4 -> Mux1/1
  Quaternions to Direction Cosine Matrix/1 -> Matrix Multiply1/1, Invert 3x3 Matrix/1
  Invert 3x3 Matrix/1 -> Matrix Multiply/1
  Product3/1 -> Gain/1
  In1/1 -> Quaternions to Direction Cosine Matrix/1

== system CthulhuFinalSimulation/Animation/q to e phi/If Action Subsystem ==
  In1 : Inport
  Action Port : ActionPort  ActionPortLabel=if(u1 ~= 0)
  Out1 : Outport
  wires:
  In1/1 -> Out1/1

== system CthulhuFinalSimulation/Animation/q to e phi/If Action Subsystem1 ==
  Action Port : ActionPort  ActionPortLabel=else
  Constant : Constant
  Out1 : Outport
  wires:
  Constant/1 -> Out1/1

== system CthulhuFinalSimulation/Buoyancy Moments1/Pitch Moment/If Action Subsystem ==
  In1 : Inport
  Action Port : ActionPort  ActionPortLabel=if(u1 ~= 0)
  Abs : Abs
  Sin : Trigonometry
  Out1 : Outport
  wires:
  In1/1 -> Abs/1
  Abs/1 -> Sin/1
  Sin/1 -> Out1/1

== system CthulhuFinalSimulation/Buoyancy Moments1/Pitch Moment/If Action Subsystem1 ==
  Action Port : ActionPort  ActionPortLabel=else
  Constant : Constant  Value=L_p/2
  Out1 : Outport
  wires:
  Constant/1 -> Out1/1

== system CthulhuFinalSimulation/Joystick Inputs1/Subsystem/throttle1 ==
  In1 : Inport
  Action Port : ActionPort  ActionPortLabel=if(u1 <= 0)
  Gain : Gain  Gain=5
  ThrustNegative : Outport  VectorParamsAs1DForOutWhenUnconnected=on
  wires:
  In1/1 -> Gain/1
  Gain/1 -> ThrustNegative/1

== system CthulhuFinalSimulation/Joystick Inputs1/Subsystem/throttle2 ==
  In2 : Inport
  Action Port : ActionPort  ActionPortLabel=else
  Gain : Gain  Gain=7.5
  ThrustPositive : Outport  VectorParamsAs1DForOutWhenUnconnected=on
  wires:
  In2/1 -> Gain/1
  Gain/1 -> ThrustPositive/1

== system CthulhuFinalSimulation/Joystick Inputs1/Subsystem2/throttle1 ==
  In1 : Inport
  Action Port : ActionPort  ActionPortLabel=if(u1 <= 0)
  Gain : Gain  Gain=5
  ThrustNegative : Outport  VectorParamsAs1DForOutWhenUnconnected=on
  wires:
  In1/1 -> Gain/1
  Gain/1 -> ThrustNegative/1

== system CthulhuFinalSimulation/Joystick Inputs1/Subsystem2/throttle2 ==
  In2 : Inport
  Action Port : ActionPort  ActionPortLabel=else
  Gain : Gain  Gain=7.5
  ThrustPositive : Outport  VectorParamsAs1DForOutWhenUnconnected=on
  wires:
  In2/1 -> Gain/1
  Gain/1 -> ThrustPositive/1

== system CthulhuFinalSimulation/Vehicle Dynamics/q propagation/If Action Subsystem ==
  Action Port : ActionPort  ActionPortLabel=if(u1 < 1e-10)
  Constant : Constant  Value=0
  Zero : Outport  InitialOutput=0
  wires:
  Constant/1 -> Zero/1

== system CthulhuFinalSimulation/Vehicle Dynamics/q propagation/If Action Subsystem1 ==
  ||B||/2 : Inport
  Action Port : ActionPort  ActionPortLabel=else
  Divide : Product  Inputs=*/
  Sin : Trigonometry
  (2/||B||)(sin(||B||/2) : Outport
  wires:
  ||B||/2/1 -> Divide/2, Sin/1
  Sin/1 -> Divide/1
  Divide/1 -> (2/||B||)(sin(||B||/2)/1
